simulink model "Lab5_Model"  (R2022a)
settings: Solver=FixedStepAuto  StartTime=0.0  StopTime=inf  FixedStep=0.001  RelTol=1e-3  EnableMultiTasking=on
undefined symbols (not defined in the file): HIL
libraries: quarc_library x3, simulink_extras x2
settings Model: SimulationMode=external  ExtModeTrigDuration=300001  Creator=ahmcmillon  LastModifiedBy=ahmcmillon
settings SolverCC: AlgebraicLoopSolver=TrustRegion  PositivePriorityOrder=on
settings DataIOCC: ReturnWorkspaceOutputs=off
settings DebuggingCC: UnconnectedInputMsg=warning  UnconnectedOutputMsg=warning  UnconnectedLineMsg=warning  PregeneratedLibrarySubsystemCodeDiagnostic=none  SFMachineParentedDataDiag=warning  ArithmeticOperatorsInVariantConditions=warning
settings SFSimCC: SimUseLocalCustomCode=off  CustomCodeUndefinedFunction=UseInterfaceOnly
settings RTWCC: Description=QUARC Win64 Target Using Toolchain  SystemTargetFile=quarc_win64.tlc  TemplateMakefile=quarc_default_tmf  RTWUseLocalCustomCode=off  Toolchain=QUARC win64 | nmake (64-bit Windows)  BuildConfiguration=Faster Runs
settings STFCustomTargetCC: TargetLangStandard=C99 (ISO)  ConcurrentExecutionCompliant=on  UseToolchainInfoCompliant=on  SystemTargetFile=quarc_win64.tlc
settings GRTTargetCC: ParMdlRefBuildCompliant=off  CompOptLevelCompliant=off  CombineOutputUpdateFcns=off  MatFileLogging=off  CPPClassGenCompliant=off  GRTInterface=on  ExtMode=on  ExtModeMexFile=quarc_comm

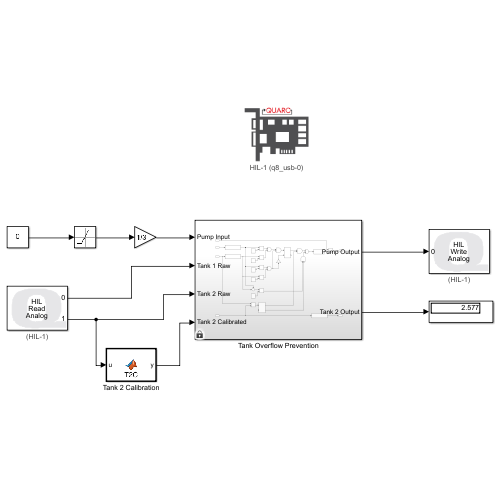
[thumbnail: Simulink's stored preview of the top-level diagram]
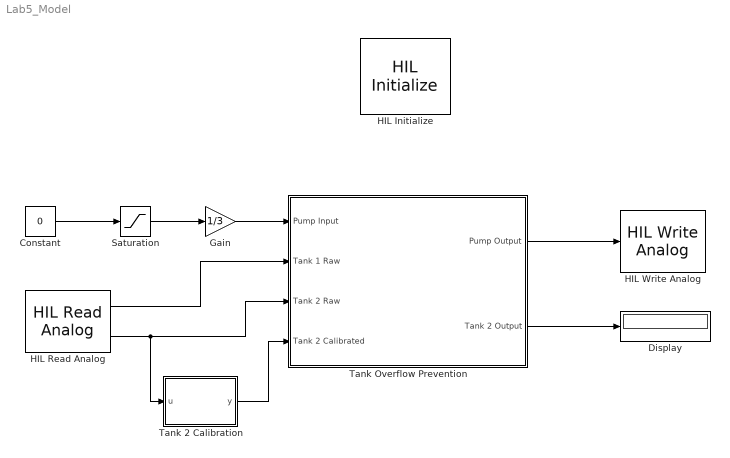
== system Lab5_Model ==
  Constant : Constant  Value=0
  Display : Display
  Gain : Gain  Gain=1/3
  HIL Initialize : quarc_library/Data Acquisition/Generic/Configuration/HIL Initialize  object_name=HIL-1  board_type=q8_usb  board_number=0  board_options=update_rate=normal;decimation=1  exclusive=off  active=on  hardware_clocks=[0:2]  clock_modes=[]  initial_clock_frequencies=[]  set_clock_params_at_start=off  set_clock_params_at_switch_in=off  set_clock_frequencies_at_start=off  set_clock_frequencies_at_switch_in=off  analog_input_channels=[0:7]  analog_input_configurations=[]  analog_input_maximums=10  analog_input_minimums=-10  set_analog_input_params_at_start=on  set_analog_input_params_at_switch_in=off  analog_output_channels=[0:7]  analog_output_maximums=10  analog_output_minimums=-10  initial_analog_outputs=[0]  final_analog_outputs=[0]  watchdog_analog_outputs=0  set_analog_output_params_at_start=on  set_analog_output_params_at_switch_in=off  set_analog_outputs_at_start=on  set_analog_outputs_at_switch_in=off  set_analog_outputs_at_terminate=on  set_analog_outputs_at_switch_out=off  set_analog_outputs_on_watchdog=off  digital_input_channels=[]  digital_output_channels=[]  digital_output_configuration=[]  initial_digital_outputs=[1]  final_digital_outputs=[1]  watchdog_digital_outputs=[1]  set_digital_output_params_at_start=off  set_digital_output_params_at_switch_in=off  set_digital_outputs_at_start=on  set_digital_outputs_at_switch_in=off  set_digital_outputs_at_terminate=on  set_digital_outputs_at_switch_out=off  set_digital_outputs_on_watchdog=off  encoder_channels=[0:7]  quadrature=[4]  encoder_filter_frequency=[]  initial_encoder_counts=[0]  set_encoder_params_at_start=on  set_encoder_params_at_switch_in=off  set_encoder_counts_at_start=on  set_encoder_counts_at_switch_in=off  pwm_channels=[0:7]  pwm_modes=0  pwm_frequency=99.532799999999995e6/4095  pwm_configuration=[0]  pwm_alignment=[0]  pwm_polarity=[1]  pwm_leading_deadband=[0]  pwm_trailing_deadband=[0]  initial_pwm_outputs=[0]  final_pwm_outputs=[0]  watchdog_pwm_outputs=[0]  set_pwm_params_at_start=on  set_pwm_params_at_switch_in=off  set_pwm_outputs_at_start=on  set_pwm_outputs_at_switch_in=off  set_pwm_outputs_at_terminate=on  set_pwm_outputs_at_switch_out=off  set_pwm_outputs_on_watchdog=off  other_output_channels=[]  initial_other_outputs=[]  final_other_outputs=[]  watchdog_other_outputs=[]  set_other_outputs_at_start=off  set_other_outputs_at_switch_in=off  set_other_outputs_at_terminate=off  set_other_outputs_at_switch_out=off  set_other_outputs_on_watchdog=off
  HIL Read Analog : quarc_library/Data Acquisition/Generic/Immediate I//O/HIL Read Analog  object_name=HIL-1  channels=[0:1]  sample_time=qc_get_step_size  active=on  vector_output=off
  HIL Write Analog : quarc_library/Data Acquisition/Generic/Immediate I//O/HIL Write Analog  object_name=HIL-1  channels=0  sample_time=-1  active=off  vector_input=off
  Saturation : Saturate  UpperLimit=22  LowerLimit=0
  Tank 2 Calibration : MATLAB Function  TreatAsAtomicUnit=on
  Tank Overflow Prevention : Subsystem
  wires:
  Gain/1 -> Tank Overflow Prevention/1(Pump Input)
  Saturation/1 -> Gain/1
  Constant/1 -> Saturation/1
  Tank Overflow Prevention/1(Pump Output) -> HIL Write Analog/1
  HIL Read Analog/1 -> Tank Overflow Prevention/2(Tank 1 Raw)
  HIL Read Analog/2 -> Tank 2 Calibration/1(u), Tank Overflow Prevention/3(Tank 2 Raw)
  Tank 2 Calibration/1(y) -> Tank Overflow Prevention/4(Tank 2 Calibrated)
  Tank Overflow Prevention/2(Tank 2 Output) -> Display/1

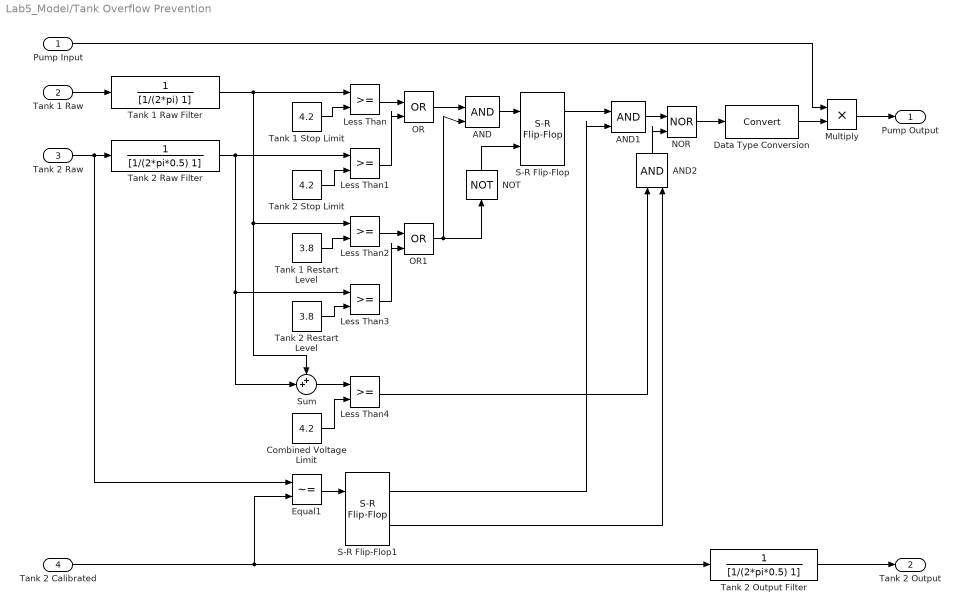
== system Lab5_Model/Tank Overflow Prevention ==
  Pump Input : Inport
  Tank 1 Raw : Inport  Port=2
  Tank 2 Raw : Inport  Port=3
  Tank 2 Calibrated : Inport  Port=4
  AND : Logic  IconShape=distinctive  AllPortsSameDT=off  OutDataTypeStr=boolean
  AND1 : Logic  IconShape=distinctive  AllPortsSameDT=off  OutDataTypeStr=boolean
  AND2 : Logic  IconShape=distinctive  AllPortsSameDT=off  OutDataTypeStr=boolean
  Combined Voltage Limit : Constant  Value=4.2
  Data Type Conversion : DataTypeConversion  OutMin=[0]  OutMax=[1]  SaturateOnIntegerOverflow=off  RndMeth=Floor
  Equal1 : RelationalOperator  Operator=~=  OutDataTypeStr=boolean  RndMeth=Simplest  InputSameDT=off
  Less Than{,1..4} (5 alike) : RelationalOperator  RndMeth=Simplest  InputSameDT=off
  Multiply : Product
  NOR : Logic  Operator=NOR  IconShape=distinctive  AllPortsSameDT=off  OutDataTypeStr=boolean
  NOT : Logic  Operator=NOT  IconShape=distinctive  AllPortsSameDT=off  OutDataTypeStr=boolean
  OR : Logic  Operator=OR  IconShape=distinctive  AllPortsSameDT=off  OutDataTypeStr=boolean
  OR1 : Logic  Operator=OR  IconShape=distinctive  AllPortsSameDT=off  OutDataTypeStr=boolean
  S-R Flip-Flop : simulink_extras/Flip Flops/S-R Flip-Flop  initial_condition=0
  S-R Flip-Flop1 : simulink_extras/Flip Flops/S-R Flip-Flop  initial_condition=0
  Sum : Sum  Inputs=++|
  Tank 1 Raw Filter : TransferFcn  Denominator=[1/(2*pi) 1]
  Tank 1 Restart Level : Constant  Value=3.8
  Tank 1 Stop Limit : Constant  Value=4.2
  Tank 2 Output Filter : TransferFcn  Denominator=[1/(2*pi*0.5) 1]
  Tank 2 Raw Filter : TransferFcn  Denominator=[1/(2*pi*0.5) 1]
  Tank 2 Restart Level : Constant  Value=3.8
  Tank 2 Stop Limit : Constant  Value=4.2
  Pump Output : Outport  VectorParamsAs1DForOutWhenUnconnected=off
  Tank 2 Output : Outport  Port=2  VectorParamsAs1DForOutWhenUnconnected=off
  wires:
  Multiply/1 -> Pump Output/1
  Pump Input/1 -> Multiply/1
  Tank 1 Stop Limit/1 -> Less Than/2
  Tank 2 Stop Limit/1 -> Less Than1/2
  Less Than/1 -> OR/1
  Less Than1/1 -> OR/2
  Data Type Conversion/1 -> Multiply/2
  Tank 1 Restart Level/1 -> Less Than2/2
  Tank 2 Restart Level/1 -> Less Than3/2
  Less Than2/1 -> OR1/1
  Less Than3/1 -> OR1/2
  OR/1 -> AND/1
  OR1/1 -> AND/2, NOT/1
  AND/1 -> S-R Flip-Flop/1
  NOT/1 -> S-R Flip-Flop/2
  Sum/1 -> Less Than4/1
  Combined Voltage Limit/1 -> Less Than4/2
  Less Than4/1 -> AND2/1
  NOR/1 -> Data Type Conversion/1
  AND2/1 -> NOR/2
  S-R Flip-Flop/1 -> AND1/1
  AND1/1 -> NOR/1
  S-R Flip-Flop1/1 -> AND1/2
  Tank 2 Calibrated/1 -> Equal1/2, Tank 2 Output Filter/1
  S-R Flip-Flop1/2 -> AND2/2
  Equal1/1 -> S-R Flip-Flop1/1
  Tank 2 Output Filter/1 -> Tank 2 Output/1
  Tank 1 Raw Filter/1 -> Sum/1, Less Than2/1, Less Than/1
  Tank 2 Raw/1 -> Tank 2 Raw Filter/1, Equal1/1
  Tank 2 Raw Filter/1 -> Sum/2, Less Than3/1, Less Than1/1
  Tank 1 Raw/1 -> Tank 1 Raw Filter/1

== matlab function Lab5_Model/Tank 2 Calibration ==
  data: u input; y output
function y = T2C(u)

y = 5.874361*u + 0.002397;
